simulink model "HAB_control"  (R2016b)
settings: Solver=VariableStepAuto  StartTime=0.0  StopTime=tf  MaxStep=1e-3  RelTol=1e-3  EnableMultiTasking=on
values from neighbouring files (symbols this model uses):
  init_speed = 100    [mainABS.m]
  k = 5e3    (= 5000)    [mainABS.m]
  lambda_init = 0    [mainABS.m]
  lambda_max = 0.35    [mainABS.m]
  lambda_min = 0.08    [mainABS.m]
  Tb_init = 0    [mainABS.m]
  Tb_max = 900    [mainABS.m]
  Tb_min = 600    [mainABS.m]
undefined symbols (not defined in the file or in its folder): auxdata
settings Model: Creator=luca  LastModifiedBy=luca
settings DataIOCC: LimitDataPoints=on
settings OptimizationCC: LifeSpan=inf
settings DebuggingCC: AllowSymbolicDim=off  SFUnexpectedBacktrackingDiag=warning  SFNoUnconditionalDefaultTransitionDiag=warning  SFExecutionAtInitializationDiag=none
settings ModelReferenceCC: PropagateSignalLabelsOutOfModel=off
settings GRTTargetCC: TargetLangStandard=C89/C90 (ANSI)
settings ConfigComp: CovMetricSettings=dw  CovHtmlReporting=on  CovSaveCumulativeToWorkspaceVar=on  CovSaveSingleToWorkspaceVar=on  CovExternalEMLEnable=off

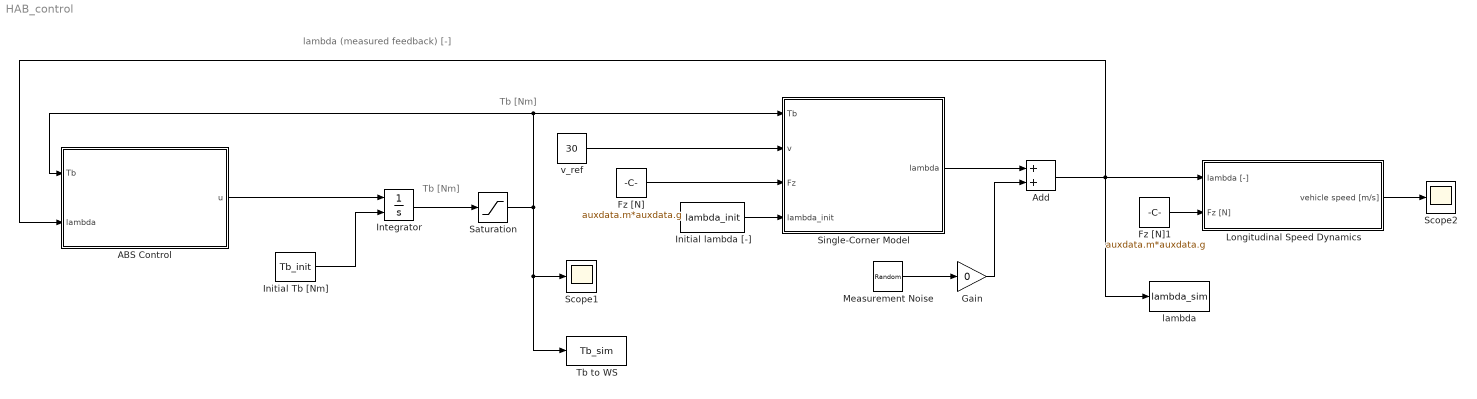
== system HAB_control ==
  note: Tb [Nm]
  note: lambda (measured feedback) [-]
  note: Tb [Nm]
  ABS Control : Stateflow chart  TreatAsAtomicUnit=on
  Add : Sum
  Fz [N] : Constant  Value=auxdata.m*auxdata.g
  Fz [N]1 : Constant  Value=auxdata.m*auxdata.g
  Gain : Gain  Gain=0
  Initial Tb [Nm] : Constant  Value=Tb_init
  Initial lambda [-] : Constant  Value=lambda_init
  Integrator : Integrator  InitialConditionSource=external
  Longitudinal Speed Dynamics : Subsystem
  Measurement Noise : RandomNumber  Variance=0.001
  Saturation : Saturate  UpperLimit=2e3  LowerLimit=0
  Scope1 : Scope
  Scope2 : Scope
  Single-Corner Model : Subsystem
      mask Display:
      | image('caliper_img.jpeg');
      | color('red');
      | port_label('output',1,'lambda [-]');
      | port_label('input',1,'Tb [Nm]');
      | port_label('input',2,'v [m/s]');
      | port_label('input',3,'Fz [N]');
      | port_label('input',4,'lambda_init [-]');
  Tb to WS : ToWorkspace  VariableName=Tb_sim  SaveFormat=Timeseries  SampleTime=-1
  lambda : ToWorkspace  VariableName=lambda_sim  SaveFormat=Timeseries  SampleTime=-1
  v_ref : Constant  Value=30
  wires:
  Initial Tb [Nm]/1 -> Integrator/2
  ABS Control/1(u) -> Integrator/1
  Fz [N]/1 -> Single-Corner Model/3(Fz)
  Initial lambda [-]/1 -> Single-Corner Model/4(lambda_init)
  Single-Corner Model/1(lambda) -> Add/1
  Measurement Noise/1 -> Gain/1
  Add/1 -> Longitudinal Speed Dynamics/1(lambda [-]), ABS Control/2(lambda), lambda/1
  Gain/1 -> Add/2
  Fz [N]1/1 -> Longitudinal Speed Dynamics/2(Fz [N])
  Longitudinal Speed Dynamics/1(vehicle speed [m/s]) -> Scope2/1
  Integrator/1 -> Saturation/1
  Saturation/1 -> ABS Control/1(Tb), Single-Corner Model/1(Tb), Tb to WS/1, Scope1/1
  v_ref/1 -> Single-Corner Model/2(v)

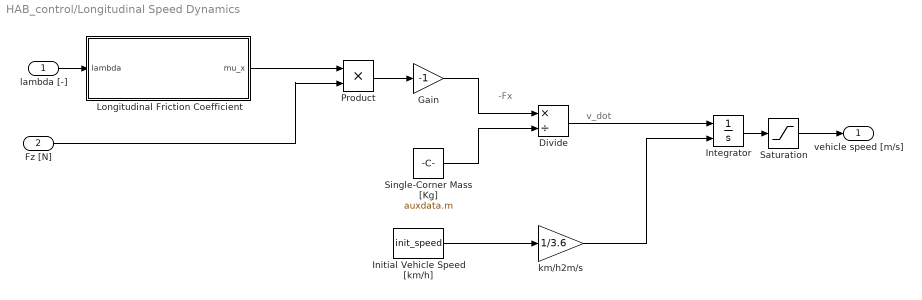
== system HAB_control/Longitudinal Speed Dynamics ==
  note: -Fx
  note: v_dot
  lambda [-] : Inport
  Fz [N] : Inport  Port=2
  Divide : Product  Inputs=*/
  Gain : Gain  Gain=-1
  Initial Vehicle Speed [km/h] : Constant  Value=init_speed
  Integrator : Integrator  InitialConditionSource=external
  Longitudinal Friction Coefficient : MATLAB Function  TreatAsAtomicUnit=on
  Product : Product
  Saturation : Saturate  UpperLimit=100  LowerLimit=0
  Single-Corner Mass [Kg] : Constant  Value=auxdata.m
  km/h2m/s : Gain  Gain=1/3.6
  vehicle speed [m/s] : Outport
  wires:
  Single-Corner Mass [Kg]/1 -> Divide/2
  Divide/1 -> Integrator/1
  km/h2m/s/1 -> Integrator/2
  Initial Vehicle Speed [km/h]/1 -> km/h2m/s/1
  Product/1 -> Gain/1
  Gain/1 -> Divide/1
  Saturation/1 -> vehicle speed [m/s]/1
  Integrator/1 -> Saturation/1
  Longitudinal Friction Coefficient/1(mu_x) -> Product/1
  Fz [N]/1 -> Product/2
  lambda [-]/1 -> Longitudinal Friction Coefficient/1(lambda)

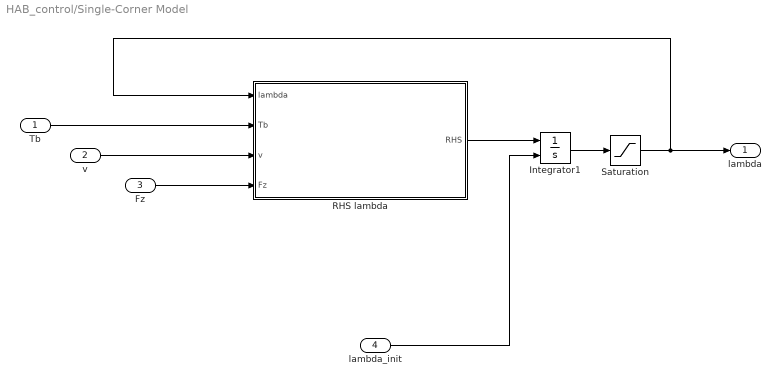
== system HAB_control/Single-Corner Model ==
  Tb : Inport
  v : Inport  Port=2
  Fz : Inport  Port=3
  lambda_init : Inport  Port=4
  Integrator1 : Integrator  InitialConditionSource=external
  RHS lambda : MATLAB Function  TreatAsAtomicUnit=on
  Saturation : Saturate  UpperLimit=0.99  LowerLimit=0
  lambda : Outport
  wires:
  Tb/1 -> RHS lambda/2(Tb)
  lambda_init/1 -> Integrator1/2
  RHS lambda/1(RHS) -> Integrator1/1
  v/1 -> RHS lambda/3(v)
  Fz/1 -> RHS lambda/4(Fz)
  Integrator1/1 -> Saturation/1
  Saturation/1 -> RHS lambda/1(lambda), lambda/1

== matlab function HAB_control/Longitudinal Speed Dynamics/Longitudinal Friction Coefficient ==
  data: lambda input; mu_x output; auxdata parameter
function mu_x = LongitudinalFrction(lambda,auxdata)
    
mu_x = burckhardt(lambda,auxdata.road_condition);

== matlab function HAB_control/Single-Corner Model/RHS lambda ==
  data: lambda input; RHS output; Tb input; v input; Fz input; auxdata parameter
function RHS = lambdaDyn(lambda,Tb,v,Fz,auxdata)
%% RHS = LAMBDADYN(lambda,Fz,road_condition)
% Right hand side of the longitudinal slip dynamics

omega = (1-lambda)*v/auxdata.r_w + eps;

Psi = (auxdata.r_w + auxdata.J/(auxdata.r_w*auxdata.m)*(1-lambda))*Fz*burckhardt(lambda,'Dry Asphalt');

RHS = -(1-lambda)/(auxdata.J*omega)*(Psi - Tb);

end

== stateflow chart HAB_control/ABS Control ==
  state State_q3
    entry: u = 0;
  state State_q2
    entry: u = -k;
  state State_q0
    entry: u = k;
  state State_q1
    entry: u = 0;
  State_q2 -> State_q3 : [Tb <= Tb_min]
  State_q3 -> State_q0 : [lambda <= lambda_min]
  (default) -> State_q0
  State_q1 -> State_q2 : [lambda >= lambda_max]
  State_q0 -> State_q1 : [Tb >= Tb_max]
  data: lambda_min parameter; Tb input; Tb_max parameter; Tb_min parameter; k parameter; lambda input; lambda_max parameter; u output
